simulink model "untitled"  (R2015b)
settings: Solver=VariableStepAuto  StartTime=0.0  StopTime=1000  RelTol=1e-3
settings Model: Creator=Pablo  LastModifiedBy=Pablo

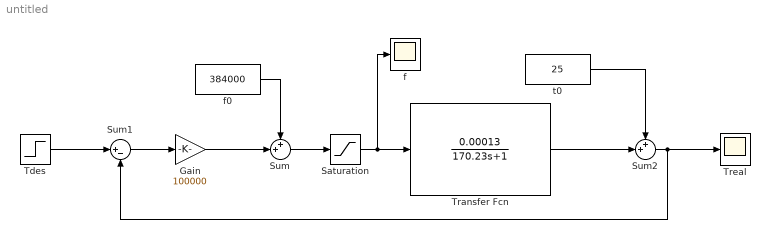
== system untitled ==
  Gain : Gain  Gain=100000
  Saturation : Saturate  UpperLimit=1700000  LowerLimit=384000
  Sum : Sum  Inputs=++|
  Sum1 : Sum  Inputs=|+-
  Sum2 : Sum  Inputs=++|
  Tdes : Step  Time=0  After=105  SampleTime=0
  Transfer Fcn : TransferFcn  Numerator=[0.00013]  Denominator=[170.23 1]
  Treal : Scope
  f : Scope
  f0 : Constant  Value=384000
  t0 : Constant  Value=25
  wires:
  Tdes/1 -> Sum1/1
  Sum1/1 -> Gain/1
  Gain/1 -> Sum/2
  f0/1 -> Sum/1
  Sum/1 -> Saturation/1
  Saturation/1 -> f/1, Transfer Fcn/1
  Sum2/1 -> Sum1/2, Treal/1
  t0/1 -> Sum2/1
  Transfer Fcn/1 -> Sum2/2
